simulink model "rectifire_single_inverter_pv1"  (R2022b)
settings: Solver=ode23tb  StartTime=0  StopTime=3  RelTol=1e-4
undefined symbols (not defined in the file): Ion, Lithium, P_100, sigbuilder_block, time_step
libraries: spsSeriesRLCBranchLib x26, spsTriangleGeneratorLib x26, slpidlib x26, spsVoltageMeasurementLib x14, spsCurrentMeasurementLib x11, spsDiodeLib x9, simulink x8, spsIGBTDiodeLib x8, spsMosfetLib x8, powerlib_extras x4, spsGroundLib x2, spsBatteryLib x2
(part 3 of 6)

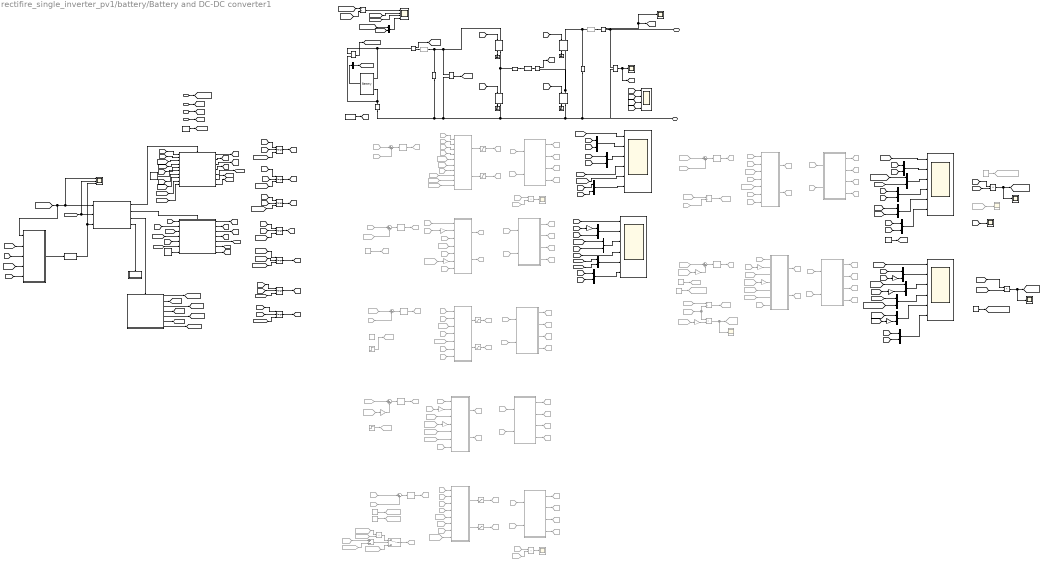
== system rectifire_single_inverter_pv1/battery/Battery and DC-DC converter1 ==
  note: Discharge in Constant Power Mode : realize by constant current
  note: Be charged in constant Current Mode
  note: Discharge in constant Current Mode
  note: Discharge in constant Voltage Mode
  note: 和开关频率同步
  note: FSBB Passivity Based Control
      | control algorithm ref: https://www.youtube.com/watch?v=5YT7cERlMrg
      | 1. Modify the topology corresponding to Gosspower hardware.
      | 1.1 add additional capacities in both input and output side
      | 1.2 add additional 2.2e-6H inductor in both input and output side to mitigate the fluctuation in constant current mode.
      | 2. Realize the constant current/voltage/Power mode in charge/discharge mode.
      |
      | Author LokiXun rongji.xun@gmail.com
  note: Be Charged in constant Voltage Mode
  note: Be Charged in Constant Power Mode : realize by constant current
  note: Constant Current/Power Transition Point
  note: Discharge in Constant Current Mode using Voltage control
  note: Charge Mode
  note: Discharge Mode
  note: Current/Voltage Protection
  Mode=Charge0/DIscharge1 : Inport
  battery_I_charge_ref : Inport  Port=2
  V_bus_ref : Inport  Port=3
  Bus_load : Inport  Port=4
  "85 volts, 100 Ah LithiumIon battery " : spsBatteryLib/Battery  BatType=Lithium-Ion  ShowTempParam=off  ThermalPreset=no  ShowAgeParam=off  NomV=85  NomQ=100  SOC=20  Batt_Tr=30  PresetModel=off  MaxQ=107.6923  MinV=83.2  FullV=115.2  Dis_rate=43.4783  R=0.08  Normal_OP=96.1538  expZone=[92.2034, 20]  current=[6.5 13 32.5]  Units=Time  Tci=20  NomT=20  T2=-30  MaxQ2=4.8  FullV2=7.1  Normal_OP2=5.655  expZone2="[6.58           1]"  Rca=0.6  ti=2000  Dp=0  Neq0=0  Tsim=1e6  Ta1=25  Qeol=5.4*0.9  Reol=0.013333*1.2  Char_age=[2.3478, 3]  Dis_age=[2.3478, 10]  N1=1500  N2=10500  N3=1000  N4=1400  Ta2=45  N5=950
      settings: LibrarySourceBlock=electricdrivelib/Extra Sources/Battery
  ActualPower1 : Scope  Commented=on
  ActualPower2 : Scope
  Battery Load : Scope  NumInputPorts=4
  BatteryCurrent1 : Scope  Commented=on
  Bus Selector : BusSelector  OutputSignals=SOC (%)
  BusPower : Scope
  C1 : spsSeriesRLCBranchLib/Series RLC Branch  LConnTagsString=__new0  RConnTagsString=__new0  BranchType=C  Resistance=0.01  Inductance=1e-3  SetiL0=off  InitialCurrent=0  Capacitance=1440e-6  Setx0=on  InitialVoltage=90  Measurements=None
  C2 : spsSeriesRLCBranchLib/Series RLC Branch  LConnTagsString=__new0  RConnTagsString=__new0  BranchType=C  Resistance=5  Inductance=1e-3  SetiL0=off  InitialCurrent=0  Capacitance=1440e-6  Setx0=on  InitialVoltage=90  Measurements=None
  Cast To Double : DataTypeConversion  OutDataTypeStr=double  SaturateOnIntegerOverflow=off  RndMeth=Floor
  Charge : Scope  NumInputPorts=6
  Charge Mixed CurrentPower1 : Subsystem  TreatAsAtomicUnit=on
  Charge Mixed CurrentPower2 : Subsystem  TreatAsAtomicUnit=on
  Constant1 : Constant  Value=time_step
  Constant10 : Constant  Value=3000
  Constant11 : Constant  Commented=on  Value=96
  Constant12 : Constant  Commented=on  Value=101
  Constant14 : Constant  Commented=on  Value=103.5
  Constant16 : Constant  Value=101
  Constant20 : Constant  Commented=on  Value=100
  Constant3 : Constant  Commented=on  Value=26
  Constant4 : Constant  Commented=on  Value=29
  Constant5 : Constant  Commented=on  Value=3000
  Current Measurement : spsCurrentMeasurementLib/Current Measurement  PhasorSimulation=off  OutputType=Complex  PSBequivalent=0
  Current Measurement1 : spsCurrentMeasurementLib/Current Measurement  PhasorSimulation=off  OutputType=Complex  PSBequivalent=0
  DM_inductor1 : spsSeriesRLCBranchLib/Series RLC Branch  Commented=through  LConnTagsString=__new0  RConnTagsString=__new0  BranchType=L  Resistance=1.0  Inductance=2.2e-6  SetiL0=off  InitialCurrent=0  Capacitance=1.0  Setx0=off  InitialVoltage=0  Measurements=None
  DM_inductor2 : spsSeriesRLCBranchLib/Series RLC Branch  Commented=through  LConnTagsString=__new0  RConnTagsString=__new0  BranchType=L  Resistance=1.0  Inductance=2.2e-6  SetiL0=off  InitialCurrent=0  Capacitance=1.0  Setx0=off  InitialVoltage=0  Measurements=None
  Discharge : Scope  NumInputPorts=6
  Discharge Const Voltage : Subsystem  TreatAsAtomicUnit=on
  Discharge+V : Scope  NumInputPorts=6
  Divide : Product  Commented=on  Inputs=*/
  Divide1 : Product  Commented=on  Inputs=*/
  Divide3 : Product  Inputs=*/
  DoNothing2 : Subsystem  TreatAsAtomicUnit=on
  From{10,24,30,32,152,168,190} (7 alike) : From  Commented=on  GotoTag=iL
  From{37..38,57..58,101,172,174,202} (8 alike) : From  Commented=on  GotoTag=i_out_ref
  From103 : From  Commented=on  GotoTag=Power_ref
  From{14,33,59,77,94,104,155,169,203} (9 alike) : From  Commented=on  GotoTag=V_battery
  From{34,41,60,74,95,107,197..198} (8 alike) : From  Commented=on  GotoTag=i_battery
  From{11..12,45,70,75,153} (6 alike) : From  Commented=on  GotoTag=VC_ref
  From{8,13,28,52..53,76,88,98,154,189,191,199} (12 alike) : From  Commented=on  GotoTag=V_bus
  From148 : From  Commented=on  GotoTag=Bus_load
  From156 : From  Commented=on  GotoTag=Bus_load
  From{18,35,54,78,157,170,200} (7 alike) : From  Commented=on  GotoTag=Ts
  From{9,36,56,79,158,171,201} (7 alike) : From  Commented=on  GotoTag=iL_ref
  From{29,31,46,55,92,96,159,192..193} (9 alike) : From  Commented=on  GotoTag=i_out
  From{16,39,49,61,64,80,173} (7 alike) : From  Commented=on  GotoTag=u1
  From{17,40,50,62,81,93,175} (7 alike) : From  Commented=on  GotoTag=u2
  From188 : From  Commented=on  GotoTag=Power_ref
  From43 : From  Commented=on  GotoTag=Power_max
  From44 : From  Commented=on  GotoTag=i_out_max_ref
  From47 : From  Commented=on  GotoTag=V_out_initial
  From48 : From  Commented=on  GotoTag=i_out_max_ref
  From51 : From  Commented=on  GotoTag=Bus_load
  Gain{,2..3,6,10..12,16..17} (9 alike) : Gain  Commented=on  Gain=-1
  Gain{7..8,14..15} (4 alike) : Gain  Gain=-1
  Goto{10,21,28..29,34,42,92} (7 alike) : Goto  Commented=on  GotoTag=S4
  Goto100 : Goto  Commented=on  GotoTag=V_power_starup
  Goto{6,12,15,17,81,88,101} (7 alike) : Goto  Commented=on  GotoTag=u1
  Goto{7,14,18,25,89,102,119} (7 alike) : Goto  Commented=on  GotoTag=u2
  Goto{8,23,31,40,77,94,103} (7 alike) : Goto  Commented=on  GotoTag=S1
  Goto{9,24,32,41,78,95,104} (7 alike) : Goto  Commented=on  GotoTag=S3
  Goto{11,22,30,33,35,43,93} (7 alike) : Goto  Commented=on  GotoTag=S2
  Goto120 : Goto  Commented=on  GotoTag=V_out_initial
  Goto126 : Goto  Commented=on  GotoTag=V_discharge_PowerMode
  Goto{19,26,46,96} (4 alike) : Goto  Commented=on  GotoTag=i_out_ref
  Goto{2,20,27,36,39,75,91} (7 alike) : Goto  Commented=on  GotoTag=iL_ref
  Goto37 : Goto  Commented=on  GotoTag=VC_ref
  Goto38 : Goto  Commented=on  GotoTag=Power_ref
  Goto76 : Goto  Commented=on  GotoTag=VC_ref
  Goto80 : Goto  Commented=on  GotoTag=i_out_max_ref
  Goto99 : Goto  Commented=on  GotoTag=Power_out
  IGBT/Diode{1..4} (4 alike) : spsIGBTDiodeLib/IGBT//Diode  Ron=1e-3  Rs=1e5  Cs=inf  Measurements=on
  IL6 : spsCurrentMeasurementLib/Current Measurement  PhasorSimulation=off  OutputType=Complex  PSBequivalent=0
  I_bus_scope : Scope
  If1 : If  NumInputs=3  IfExpression="u3 == 0 & u1 == 1  & u2 > 10"  ElseIfExpressions=u3 == 0 & u1 == 0 & u2 < 95, u3==1
  MATLAB Function : MATLAB Function  Commented=on  TreatAsAtomicUnit=on
  MATLAB Function1 : MATLAB Function  Commented=on  TreatAsAtomicUnit=on
  MATLAB Function2 : MATLAB Function  Commented=on  TreatAsAtomicUnit=on
  MATLAB Function3 : MATLAB Function  Commented=on  TreatAsAtomicUnit=on
  MATLAB Function4 : MATLAB Function  TreatAsAtomicUnit=on
  MATLAB Function5 : MATLAB Function  Commented=on  TreatAsAtomicUnit=on
  MATLAB Function6 : MATLAB Function  Commented=on  TreatAsAtomicUnit=on
  MATLAB Function7 : MATLAB Function  Commented=on  TreatAsAtomicUnit=on
  Minus : Sum  Commented=on  Inputs=+-
  Modulation : Subsystem  Commented=on
  Modulation1 : Subsystem  Commented=on
  Modulation2 : Subsystem  Commented=on
  Modulation3 : Subsystem  Commented=on
  Modulation4 : Subsystem  Commented=on
  Modulation5 : Subsystem  Commented=on
  Modulation6 : Subsystem  Commented=on
  Mux{,1..4,9..21} (18 alike) : Mux  Inputs=2
  PID Controller1 : slpidlib/PID Controller  Commented=on  Controller=PI  Form=Parallel  TimeDomain=Continuous-time  UseExternalTs=off  SampleTime=-1  IntegratorMethod=Forward Euler  FilterMethod=Forward Euler  ControllerParametersSource=internal  P=6.7500  I=8.1000e+03 * 2  UseKiTs=on  D=0  N=100  UseFilter=on  TunerSelectOption=Transfer Function Based (PID Tuner App)  InitialConditionSource=internal  InitialConditionForIntegrator=0  InitialConditionForFilter=0  DifferentiatorICPrevScaledInput=0  ExternalReset=none  TrackingMode=off  Kt=1  LimitOutput=on  SatLimitsSource=internal  UpperSaturationLimit=50  LowerSaturationLimit=-10  LinearizeAsGain=on  AntiWindupMode=none  Kb=1  LimitIntegrator=off  UpperIntegratorSaturationLimit=inf  LowerIntegratorSaturationLimit=-inf  POutMin=[]  POutMax=[]  IOutMin=[]  IOutMax=[]  DOutMin=[]  DOutMax=[]  NOutMin=[]  NOutMax=[]  SumOutMin=[]  SumOutMax=[]  SaturationOutMin=[]  SaturationOutMax=[]  PParamMin=[]  PParamMax=[]  IParamMin=[]  IParamMax=[]  DParamMin=[]  DParamMax=[]  NParamMin=[]  NParamMax=[]  KbParamMin=[]  KbParamMax=[]  KtParamMin=[]  KtParamMax=[]  KbOutMin=[]  KbOutMax=[]  KtOutMin=[]  KtOutMax=[]  IntegratorOutMin=[]  IntegratorOutMax=[]  FilterOutMin=[]  FilterOutMax=[]  SumI1OutMin=[]  SumI1OutMax=[]  SumI2OutMin=[]  SumI2OutMax=[]  SumI3OutMin=[]  SumI3OutMax=[]  SumI4OutMin=[]  SumI4OutMax=[]  SumDOutMin=[]  SumDOutMax=[]  DifferentiatorOutMin=[]  DifferentiatorOutMax=[]  FilterDiffOutCoefMin=[]  FilterDiffOutCoefMax=[]  ReciprocalOutMin=[]  ReciprocalOutMax=[]  SumDenOutMin=[]  SumDenOutMax=[]  SumNumOutMin=[]  SumNumOutMax=[]  DivideOutMin=[]  DivideOutMax=[]  UdiffTsProdOutMin=[]  UdiffTsProdOutMax=[]  NTsProdOutMin=[]  NTsProdOutMax=[]  UintegralTsProdOutMin=[]  UintegralTsProdOutMax=[]  UngainTsProdOutMin=[]  UngainTsProdOutMax=[]  ClampingZeroOutDataTypeStr=Inherit: Inherit via back propagation  ClampingZeroOutMin=[]  ClampingZeroOutMax=[]  FilterDenConstantOutDataTypeStr=Inherit: Inherit via back propagation  FilterDenConstantOutMin=[]  FilterDenConstantOutMax=[]  PCopyOutDataTypeStr=Inherit: Inherit via back propagation  PCopyOutMin=[]  PCopyOutMax=[]  NCopyOutDataTypeStr=Inherit: Inherit via back propagation  NCopyOutMin=[]  NCopyOutMax=[]  IntegratorContinuousStateAttributes=''  IntegratorStateMustResolveToSignalObject=off  IntegratorRTWStateStorageClass=Auto  FilterContinuousStateAttributes=''  FilterStateMustResolveToSignalObject=off  FilterRTWStateStorageClass=Auto  ParallelPVariant=InternalParameters  IdealPVariant=Disabled  IVariant=InternalParameters  DVariant=Disabled  IntegratorVariant=Continuous  SatVariant=Enabled  AWVariant=Passthrough  PCopyVariant=Disabled  TRVariant=Disabled  FdbkBlocksVariant=Forward  IdealPFdbkVariant=Disabled  SatFdbkVariant=Disabled  DerivativeFilterVariant=Disabled  NVariant=Disabled  NCopyVariant=Disabled_SignalSpec  FilterICVariant=Disabled  IntegratorICVariant=InternalICs  ExternalResetVariant=Disabled  TRSumVariant=Passthrough  SumFdbkVariant=Disabled  SumVariant=Sum_PI  TsampFilterVariant=InternalTs  TsampNgainVariant=Passthrough  TsampIntegralVariant=Passthrough  ExternalSaturationOutDataTypeStr=Inherit: Same as second input
  PID Controller2 : slpidlib/PID Controller  Commented=on  Controller=PI  Form=Parallel  TimeDomain=Continuous-time  UseExternalTs=off  SampleTime=-1  IntegratorMethod=Forward Euler  FilterMethod=Forward Euler  ControllerParametersSource=internal  P=45 * 2  I=1.3361e+05 /25  UseKiTs=on  D=0  N=100  UseFilter=on  TunerSelectOption=Frequency Response Based  InitialConditionSource=internal  InitialConditionForIntegrator=0  InitialConditionForFilter=0  DifferentiatorICPrevScaledInput=0  ExternalReset=none  TrackingMode=off  Kt=1  LimitOutput=on  SatLimitsSource=internal  UpperSaturationLimit=50  LowerSaturationLimit=-10  LinearizeAsGain=on  AntiWindupMode=none  Kb=1  LimitIntegrator=off  UpperIntegratorSaturationLimit=inf  LowerIntegratorSaturationLimit=-inf  POutMin=[]  POutMax=[]  IOutMin=[]  IOutMax=[]  DOutMin=[]  DOutMax=[]  NOutMin=[]  NOutMax=[]  SumOutMin=[]  SumOutMax=[]  SaturationOutMin=[]  SaturationOutMax=[]  PParamMin=[]  PParamMax=[]  IParamMin=[]  IParamMax=[]  DParamMin=[]  DParamMax=[]  NParamMin=[]  NParamMax=[]  KbParamMin=[]  KbParamMax=[]  KtParamMin=[]  KtParamMax=[]  KbOutMin=[]  KbOutMax=[]  KtOutMin=[]  KtOutMax=[]  IntegratorOutMin=[]  IntegratorOutMax=[]  FilterOutMin=[]  FilterOutMax=[]  SumI1OutMin=[]  SumI1OutMax=[]  SumI2OutMin=[]  SumI2OutMax=[]  SumI3OutMin=[]  SumI3OutMax=[]  SumI4OutMin=[]  SumI4OutMax=[]  SumDOutMin=[]  SumDOutMax=[]  DifferentiatorOutMin=[]  DifferentiatorOutMax=[]  FilterDiffOutCoefMin=[]  FilterDiffOutCoefMax=[]  ReciprocalOutMin=[]  ReciprocalOutMax=[]  SumDenOutMin=[]  SumDenOutMax=[]  SumNumOutMin=[]  SumNumOutMax=[]  DivideOutMin=[]  DivideOutMax=[]  UdiffTsProdOutMin=[]  UdiffTsProdOutMax=[]  NTsProdOutMin=[]  NTsProdOutMax=[]  UintegralTsProdOutMin=[]  UintegralTsProdOutMax=[]  UngainTsProdOutMin=[]  UngainTsProdOutMax=[]  ClampingZeroOutDataTypeStr=Inherit: Inherit via back propagation  ClampingZeroOutMin=[]  ClampingZeroOutMax=[]  FilterDenConstantOutDataTypeStr=Inherit: Inherit via back propagation  FilterDenConstantOutMin=[]  FilterDenConstantOutMax=[]  PCopyOutDataTypeStr=Inherit: Inherit via back propagation  PCopyOutMin=[]  PCopyOutMax=[]  NCopyOutDataTypeStr=Inherit: Inherit via back propagation  NCopyOutMin=[]  NCopyOutMax=[]  IntegratorContinuousStateAttributes=''  IntegratorStateMustResolveToSignalObject=off  IntegratorRTWStateStorageClass=Auto  FilterContinuousStateAttributes=''  FilterStateMustResolveToSignalObject=off  FilterRTWStateStorageClass=Auto  ParallelPVariant=InternalParameters  IdealPVariant=Disabled  IVariant=InternalParameters  DVariant=Disabled  IntegratorVariant=Continuous  SatVariant=Enabled  AWVariant=Passthrough  PCopyVariant=Disabled  TRVariant=Disabled  FdbkBlocksVariant=Forward  IdealPFdbkVariant=Disabled  SatFdbkVariant=Disabled  DerivativeFilterVariant=Disabled  NVariant=Disabled  NCopyVariant=Disabled_SignalSpec  FilterICVariant=Disabled  IntegratorICVariant=InternalICs  ExternalResetVariant=Disabled  TRSumVariant=Passthrough  SumFdbkVariant=Disabled  SumVariant=Sum_PI  TsampFilterVariant=InternalTs  TsampNgainVariant=Passthrough  TsampIntegralVariant=Passthrough  ExternalSaturationOutDataTypeStr=Inherit: Same as second input
  PID Controller3 : slpidlib/PID Controller  Commented=on  Controller=PI  Form=Parallel  TimeDomain=Continuous-time  UseExternalTs=off  SampleTime=-1  IntegratorMethod=Forward Euler  FilterMethod=Forward Euler  ControllerParametersSource=internal  P=6.7500  I=8.1000e+03 * 2  UseKiTs=on  D=0  N=100  UseFilter=on  TunerSelectOption=Transfer Function Based (PID Tuner App)  InitialConditionSource=internal  InitialConditionForIntegrator=0  InitialConditionForFilter=0  DifferentiatorICPrevScaledInput=0  ExternalReset=none  TrackingMode=off  Kt=1  LimitOutput=on  SatLimitsSource=internal  UpperSaturationLimit=50  LowerSaturationLimit=-10  LinearizeAsGain=on  AntiWindupMode=none  Kb=1  LimitIntegrator=off  UpperIntegratorSaturationLimit=inf  LowerIntegratorSaturationLimit=-inf  POutMin=[]  POutMax=[]  IOutMin=[]  IOutMax=[]  DOutMin=[]  DOutMax=[]  NOutMin=[]  NOutMax=[]  SumOutMin=[]  SumOutMax=[]  SaturationOutMin=[]  SaturationOutMax=[]  PParamMin=[]  PParamMax=[]  IParamMin=[]  IParamMax=[]  DParamMin=[]  DParamMax=[]  NParamMin=[]  NParamMax=[]  KbParamMin=[]  KbParamMax=[]  KtParamMin=[]  KtParamMax=[]  KbOutMin=[]  KbOutMax=[]  KtOutMin=[]  KtOutMax=[]  IntegratorOutMin=[]  IntegratorOutMax=[]  FilterOutMin=[]  FilterOutMax=[]  SumI1OutMin=[]  SumI1OutMax=[]  SumI2OutMin=[]  SumI2OutMax=[]  SumI3OutMin=[]  SumI3OutMax=[]  SumI4OutMin=[]  SumI4OutMax=[]  SumDOutMin=[]  SumDOutMax=[]  DifferentiatorOutMin=[]  DifferentiatorOutMax=[]  FilterDiffOutCoefMin=[]  FilterDiffOutCoefMax=[]  ReciprocalOutMin=[]  ReciprocalOutMax=[]  SumDenOutMin=[]  SumDenOutMax=[]  SumNumOutMin=[]  SumNumOutMax=[]  DivideOutMin=[]  DivideOutMax=[]  UdiffTsProdOutMin=[]  UdiffTsProdOutMax=[]  NTsProdOutMin=[]  NTsProdOutMax=[]  UintegralTsProdOutMin=[]  UintegralTsProdOutMax=[]  UngainTsProdOutMin=[]  UngainTsProdOutMax=[]  ClampingZeroOutDataTypeStr=Inherit: Inherit via back propagation  ClampingZeroOutMin=[]  ClampingZeroOutMax=[]  FilterDenConstantOutDataTypeStr=Inherit: Inherit via back propagation  FilterDenConstantOutMin=[]  FilterDenConstantOutMax=[]  PCopyOutDataTypeStr=Inherit: Inherit via back propagation  PCopyOutMin=[]  PCopyOutMax=[]  NCopyOutDataTypeStr=Inherit: Inherit via back propagation  NCopyOutMin=[]  NCopyOutMax=[]  IntegratorContinuousStateAttributes=''  IntegratorStateMustResolveToSignalObject=off  IntegratorRTWStateStorageClass=Auto  FilterContinuousStateAttributes=''  FilterStateMustResolveToSignalObject=off  FilterRTWStateStorageClass=Auto  ParallelPVariant=InternalParameters  IdealPVariant=Disabled  IVariant=InternalParameters  DVariant=Disabled  IntegratorVariant=Continuous  SatVariant=Enabled  AWVariant=Passthrough  PCopyVariant=Disabled  TRVariant=Disabled  FdbkBlocksVariant=Forward  IdealPFdbkVariant=Disabled  SatFdbkVariant=Disabled  DerivativeFilterVariant=Disabled  NVariant=Disabled  NCopyVariant=Disabled_SignalSpec  FilterICVariant=Disabled  IntegratorICVariant=InternalICs  ExternalResetVariant=Disabled  TRSumVariant=Passthrough  SumFdbkVariant=Disabled  SumVariant=Sum_PI  TsampFilterVariant=InternalTs  TsampNgainVariant=Passthrough  TsampIntegralVariant=Passthrough  ExternalSaturationOutDataTypeStr=Inherit: Same as second input
  PID Controller4 : slpidlib/PID Controller  Commented=on  Controller=PI  Form=Parallel  TimeDomain=Continuous-time  UseExternalTs=off  SampleTime=-1  IntegratorMethod=Forward Euler  FilterMethod=Forward Euler  ControllerParametersSource=internal  P=15  I=1000  UseKiTs=on  D=0  N=100  UseFilter=on  TunerSelectOption=Transfer Function Based (PID Tuner App)  InitialConditionSource=internal  InitialConditionForIntegrator=0  InitialConditionForFilter=0  DifferentiatorICPrevScaledInput=0  ExternalReset=none  TrackingMode=off  Kt=1  LimitOutput=on  SatLimitsSource=internal  UpperSaturationLimit=50  LowerSaturationLimit=-10  LinearizeAsGain=on  AntiWindupMode=none  Kb=1  LimitIntegrator=off  UpperIntegratorSaturationLimit=inf  LowerIntegratorSaturationLimit=-inf  POutMin=[]  POutMax=[]  IOutMin=[]  IOutMax=[]  DOutMin=[]  DOutMax=[]  NOutMin=[]  NOutMax=[]  SumOutMin=[]  SumOutMax=[]  SaturationOutMin=[]  SaturationOutMax=[]  PParamMin=[]  PParamMax=[]  IParamMin=[]  IParamMax=[]  DParamMin=[]  DParamMax=[]  NParamMin=[]  NParamMax=[]  KbParamMin=[]  KbParamMax=[]  KtParamMin=[]  KtParamMax=[]  KbOutMin=[]  KbOutMax=[]  KtOutMin=[]  KtOutMax=[]  IntegratorOutMin=[]  IntegratorOutMax=[]  FilterOutMin=[]  FilterOutMax=[]  SumI1OutMin=[]  SumI1OutMax=[]  SumI2OutMin=[]  SumI2OutMax=[]  SumI3OutMin=[]  SumI3OutMax=[]  SumI4OutMin=[]  SumI4OutMax=[]  SumDOutMin=[]  SumDOutMax=[]  DifferentiatorOutMin=[]  DifferentiatorOutMax=[]  FilterDiffOutCoefMin=[]  FilterDiffOutCoefMax=[]  ReciprocalOutMin=[]  ReciprocalOutMax=[]  SumDenOutMin=[]  SumDenOutMax=[]  SumNumOutMin=[]  SumNumOutMax=[]  DivideOutMin=[]  DivideOutMax=[]  UdiffTsProdOutMin=[]  UdiffTsProdOutMax=[]  NTsProdOutMin=[]  NTsProdOutMax=[]  UintegralTsProdOutMin=[]  UintegralTsProdOutMax=[]  UngainTsProdOutMin=[]  UngainTsProdOutMax=[]  ClampingZeroOutDataTypeStr=Inherit: Inherit via back propagation  ClampingZeroOutMin=[]  ClampingZeroOutMax=[]  FilterDenConstantOutDataTypeStr=Inherit: Inherit via back propagation  FilterDenConstantOutMin=[]  FilterDenConstantOutMax=[]  PCopyOutDataTypeStr=Inherit: Inherit via back propagation  PCopyOutMin=[]  PCopyOutMax=[]  NCopyOutDataTypeStr=Inherit: Inherit via back propagation  NCopyOutMin=[]  NCopyOutMax=[]  IntegratorContinuousStateAttributes=''  IntegratorStateMustResolveToSignalObject=off  IntegratorRTWStateStorageClass=Auto  FilterContinuousStateAttributes=''  FilterStateMustResolveToSignalObject=off  FilterRTWStateStorageClass=Auto  ParallelPVariant=InternalParameters  IdealPVariant=Disabled  IVariant=InternalParameters  DVariant=Disabled  IntegratorVariant=Continuous  SatVariant=Enabled  AWVariant=Passthrough  PCopyVariant=Disabled  TRVariant=Disabled  FdbkBlocksVariant=Forward  IdealPFdbkVariant=Disabled  SatFdbkVariant=Disabled  DerivativeFilterVariant=Disabled  NVariant=Disabled  NCopyVariant=Disabled_SignalSpec  FilterICVariant=Disabled  IntegratorICVariant=InternalICs  ExternalResetVariant=Disabled  TRSumVariant=Passthrough  SumFdbkVariant=Disabled  SumVariant=Sum_PI  TsampFilterVariant=InternalTs  TsampNgainVariant=Passthrough  TsampIntegralVariant=Passthrough  ExternalSaturationOutDataTypeStr=Inherit: Same as second input
  PID Controller5 : slpidlib/PID Controller  Commented=on  Controller=PI  Form=Parallel  TimeDomain=Continuous-time  UseExternalTs=off  SampleTime=-1  IntegratorMethod=Forward Euler  FilterMethod=Forward Euler  ControllerParametersSource=internal  P=15  I=1000  UseKiTs=on  D=0  N=100  UseFilter=on  TunerSelectOption=Transfer Function Based (PID Tuner App)  InitialConditionSource=internal  InitialConditionForIntegrator=0  InitialConditionForFilter=0  DifferentiatorICPrevScaledInput=0  ExternalReset=none  TrackingMode=off  Kt=1  LimitOutput=on  SatLimitsSource=internal  UpperSaturationLimit=50  LowerSaturationLimit=-10  LinearizeAsGain=on  AntiWindupMode=none  Kb=1  LimitIntegrator=off  UpperIntegratorSaturationLimit=inf  LowerIntegratorSaturationLimit=-inf  POutMin=[]  POutMax=[]  IOutMin=[]  IOutMax=[]  DOutMin=[]  DOutMax=[]  NOutMin=[]  NOutMax=[]  SumOutMin=[]  SumOutMax=[]  SaturationOutMin=[]  SaturationOutMax=[]  PParamMin=[]  PParamMax=[]  IParamMin=[]  IParamMax=[]  DParamMin=[]  DParamMax=[]  NParamMin=[]  NParamMax=[]  KbParamMin=[]  KbParamMax=[]  KtParamMin=[]  KtParamMax=[]  KbOutMin=[]  KbOutMax=[]  KtOutMin=[]  KtOutMax=[]  IntegratorOutMin=[]  IntegratorOutMax=[]  FilterOutMin=[]  FilterOutMax=[]  SumI1OutMin=[]  SumI1OutMax=[]  SumI2OutMin=[]  SumI2OutMax=[]  SumI3OutMin=[]  SumI3OutMax=[]  SumI4OutMin=[]  SumI4OutMax=[]  SumDOutMin=[]  SumDOutMax=[]  DifferentiatorOutMin=[]  DifferentiatorOutMax=[]  FilterDiffOutCoefMin=[]  FilterDiffOutCoefMax=[]  ReciprocalOutMin=[]  ReciprocalOutMax=[]  SumDenOutMin=[]  SumDenOutMax=[]  SumNumOutMin=[]  SumNumOutMax=[]  DivideOutMin=[]  DivideOutMax=[]  UdiffTsProdOutMin=[]  UdiffTsProdOutMax=[]  NTsProdOutMin=[]  NTsProdOutMax=[]  UintegralTsProdOutMin=[]  UintegralTsProdOutMax=[]  UngainTsProdOutMin=[]  UngainTsProdOutMax=[]  ClampingZeroOutDataTypeStr=Inherit: Inherit via back propagation  ClampingZeroOutMin=[]  ClampingZeroOutMax=[]  FilterDenConstantOutDataTypeStr=Inherit: Inherit via back propagation  FilterDenConstantOutMin=[]  FilterDenConstantOutMax=[]  PCopyOutDataTypeStr=Inherit: Inherit via back propagation  PCopyOutMin=[]  PCopyOutMax=[]  NCopyOutDataTypeStr=Inherit: Inherit via back propagation  NCopyOutMin=[]  NCopyOutMax=[]  IntegratorContinuousStateAttributes=''  IntegratorStateMustResolveToSignalObject=off  IntegratorRTWStateStorageClass=Auto  FilterContinuousStateAttributes=''  FilterStateMustResolveToSignalObject=off  FilterRTWStateStorageClass=Auto  ParallelPVariant=InternalParameters  IdealPVariant=Disabled  IVariant=InternalParameters  DVariant=Disabled  IntegratorVariant=Continuous  SatVariant=Enabled  AWVariant=Passthrough  PCopyVariant=Disabled  TRVariant=Disabled  FdbkBlocksVariant=Forward  IdealPFdbkVariant=Disabled  SatFdbkVariant=Disabled  DerivativeFilterVariant=Disabled  NVariant=Disabled  NCopyVariant=Disabled_SignalSpec  FilterICVariant=Disabled  IntegratorICVariant=InternalICs  ExternalResetVariant=Disabled  TRSumVariant=Passthrough  SumFdbkVariant=Disabled  SumVariant=Sum_PI  TsampFilterVariant=InternalTs  TsampNgainVariant=Passthrough  TsampIntegralVariant=Passthrough  ExternalSaturationOutDataTypeStr=Inherit: Same as second input
  PID Controller6 : slpidlib/PID Controller  Commented=on  Controller=PI  Form=Parallel  TimeDomain=Continuous-time  UseExternalTs=off  SampleTime=-1  IntegratorMethod=Forward Euler  FilterMethod=Forward Euler  ControllerParametersSource=internal  P=15  I=1000  UseKiTs=on  D=0  N=100  UseFilter=on  TunerSelectOption=Transfer Function Based (PID Tuner App)  InitialConditionSource=internal  InitialConditionForIntegrator=0  InitialConditionForFilter=0  DifferentiatorICPrevScaledInput=0  ExternalReset=none  TrackingMode=off  Kt=1  LimitOutput=on  SatLimitsSource=internal  UpperSaturationLimit=50  LowerSaturationLimit=-10  LinearizeAsGain=on  AntiWindupMode=none  Kb=1  LimitIntegrator=off  UpperIntegratorSaturationLimit=inf  LowerIntegratorSaturationLimit=-inf  POutMin=[]  POutMax=[]  IOutMin=[]  IOutMax=[]  DOutMin=[]  DOutMax=[]  NOutMin=[]  NOutMax=[]  SumOutMin=[]  SumOutMax=[]  SaturationOutMin=[]  SaturationOutMax=[]  PParamMin=[]  PParamMax=[]  IParamMin=[]  IParamMax=[]  DParamMin=[]  DParamMax=[]  NParamMin=[]  NParamMax=[]  KbParamMin=[]  KbParamMax=[]  KtParamMin=[]  KtParamMax=[]  KbOutMin=[]  KbOutMax=[]  KtOutMin=[]  KtOutMax=[]  IntegratorOutMin=[]  IntegratorOutMax=[]  FilterOutMin=[]  FilterOutMax=[]  SumI1OutMin=[]  SumI1OutMax=[]  SumI2OutMin=[]  SumI2OutMax=[]  SumI3OutMin=[]  SumI3OutMax=[]  SumI4OutMin=[]  SumI4OutMax=[]  SumDOutMin=[]  SumDOutMax=[]  DifferentiatorOutMin=[]  DifferentiatorOutMax=[]  FilterDiffOutCoefMin=[]  FilterDiffOutCoefMax=[]  ReciprocalOutMin=[]  ReciprocalOutMax=[]  SumDenOutMin=[]  SumDenOutMax=[]  SumNumOutMin=[]  SumNumOutMax=[]  DivideOutMin=[]  DivideOutMax=[]  UdiffTsProdOutMin=[]  UdiffTsProdOutMax=[]  NTsProdOutMin=[]  NTsProdOutMax=[]  UintegralTsProdOutMin=[]  UintegralTsProdOutMax=[]  UngainTsProdOutMin=[]  UngainTsProdOutMax=[]  ClampingZeroOutDataTypeStr=Inherit: Inherit via back propagation  ClampingZeroOutMin=[]  ClampingZeroOutMax=[]  FilterDenConstantOutDataTypeStr=Inherit: Inherit via back propagation  FilterDenConstantOutMin=[]  FilterDenConstantOutMax=[]  PCopyOutDataTypeStr=Inherit: Inherit via back propagation  PCopyOutMin=[]  PCopyOutMax=[]  NCopyOutDataTypeStr=Inherit: Inherit via back propagation  NCopyOutMin=[]  NCopyOutMax=[]  IntegratorContinuousStateAttributes=''  IntegratorStateMustResolveToSignalObject=off  IntegratorRTWStateStorageClass=Auto  FilterContinuousStateAttributes=''  FilterStateMustResolveToSignalObject=off  FilterRTWStateStorageClass=Auto  ParallelPVariant=InternalParameters  IdealPVariant=Disabled  IVariant=InternalParameters  DVariant=Disabled  IntegratorVariant=Continuous  SatVariant=Enabled  AWVariant=Passthrough  PCopyVariant=Disabled  TRVariant=Disabled  FdbkBlocksVariant=Forward  IdealPFdbkVariant=Disabled  SatFdbkVariant=Disabled  DerivativeFilterVariant=Disabled  NVariant=Disabled  NCopyVariant=Disabled_SignalSpec  FilterICVariant=Disabled  IntegratorICVariant=InternalICs  ExternalResetVariant=Disabled  TRSumVariant=Passthrough  SumFdbkVariant=Disabled  SumVariant=Sum_PI  TsampFilterVariant=InternalTs  TsampNgainVariant=Passthrough  TsampIntegralVariant=Passthrough  ExternalSaturationOutDataTypeStr=Inherit: Same as second input
  PID Controller7 : slpidlib/PID Controller  Commented=on  Controller=PI  Form=Parallel  TimeDomain=Continuous-time  UseExternalTs=off  SampleTime=-1  IntegratorMethod=Forward Euler  FilterMethod=Forward Euler  ControllerParametersSource=internal  P=45 * 2  I=1.3361e+05 /25  UseKiTs=on  D=0  N=100  UseFilter=on  TunerSelectOption=Transfer Function Based (PID Tuner App)  InitialConditionSource=internal  InitialConditionForIntegrator=0  InitialConditionForFilter=0  DifferentiatorICPrevScaledInput=0  ExternalReset=none  TrackingMode=off  Kt=1  LimitOutput=on  SatLimitsSource=internal  UpperSaturationLimit=50  LowerSaturationLimit=-10  LinearizeAsGain=on  AntiWindupMode=none  Kb=1  LimitIntegrator=off  UpperIntegratorSaturationLimit=inf  LowerIntegratorSaturationLimit=-inf  POutMin=[]  POutMax=[]  IOutMin=[]  IOutMax=[]  DOutMin=[]  DOutMax=[]  NOutMin=[]  NOutMax=[]  SumOutMin=[]  SumOutMax=[]  SaturationOutMin=[]  SaturationOutMax=[]  PParamMin=[]  PParamMax=[]  IParamMin=[]  IParamMax=[]  DParamMin=[]  DParamMax=[]  NParamMin=[]  NParamMax=[]  KbParamMin=[]  KbParamMax=[]  KtParamMin=[]  KtParamMax=[]  KbOutMin=[]  KbOutMax=[]  KtOutMin=[]  KtOutMax=[]  IntegratorOutMin=[]  IntegratorOutMax=[]  FilterOutMin=[]  FilterOutMax=[]  SumI1OutMin=[]  SumI1OutMax=[]  SumI2OutMin=[]  SumI2OutMax=[]  SumI3OutMin=[]  SumI3OutMax=[]  SumI4OutMin=[]  SumI4OutMax=[]  SumDOutMin=[]  SumDOutMax=[]  DifferentiatorOutMin=[]  DifferentiatorOutMax=[]  FilterDiffOutCoefMin=[]  FilterDiffOutCoefMax=[]  ReciprocalOutMin=[]  ReciprocalOutMax=[]  SumDenOutMin=[]  SumDenOutMax=[]  SumNumOutMin=[]  SumNumOutMax=[]  DivideOutMin=[]  DivideOutMax=[]  UdiffTsProdOutMin=[]  UdiffTsProdOutMax=[]  NTsProdOutMin=[]  NTsProdOutMax=[]  UintegralTsProdOutMin=[]  UintegralTsProdOutMax=[]  UngainTsProdOutMin=[]  UngainTsProdOutMax=[]  ClampingZeroOutDataTypeStr=Inherit: Inherit via back propagation  ClampingZeroOutMin=[]  ClampingZeroOutMax=[]  FilterDenConstantOutDataTypeStr=Inherit: Inherit via back propagation  FilterDenConstantOutMin=[]  FilterDenConstantOutMax=[]  PCopyOutDataTypeStr=Inherit: Inherit via back propagation  PCopyOutMin=[]  PCopyOutMax=[]  NCopyOutDataTypeStr=Inherit: Inherit via back propagation  NCopyOutMin=[]  NCopyOutMax=[]  IntegratorContinuousStateAttributes=''  IntegratorStateMustResolveToSignalObject=off  IntegratorRTWStateStorageClass=Auto  FilterContinuousStateAttributes=''  FilterStateMustResolveToSignalObject=off  FilterRTWStateStorageClass=Auto  ParallelPVariant=InternalParameters  IdealPVariant=Disabled  IVariant=InternalParameters  DVariant=Disabled  IntegratorVariant=Continuous  SatVariant=Enabled  AWVariant=Passthrough  PCopyVariant=Disabled  TRVariant=Disabled  FdbkBlocksVariant=Forward  IdealPFdbkVariant=Disabled  SatFdbkVariant=Disabled  DerivativeFilterVariant=Disabled  NVariant=Disabled  NCopyVariant=Disabled_SignalSpec  FilterICVariant=Disabled  IntegratorICVariant=InternalICs  ExternalResetVariant=Disabled  TRSumVariant=Passthrough  SumFdbkVariant=Disabled  SumVariant=Sum_PI  TsampFilterVariant=InternalTs  TsampNgainVariant=Passthrough  TsampIntegralVariant=Passthrough  ExternalSaturationOutDataTypeStr=Inherit: Same as second input
  Power : Scope  Commented=on
  Power1 : Scope  Commented=on
  Product{,2..3,5} (4 alike) : Product  Commented=on
  Product1 : Product
  Product4 : Product
  R_battery : spsSeriesRLCBranchLib/Series RLC Branch  LConnTagsString=__new0  RConnTagsString=__new0  BranchType=R  Resistance=0.1  Inductance=1e-3  SetiL0=off  InitialCurrent=0  Capacitance=1440e-6  Setx0=off  InitialVoltage=80  Measurements=None
  S1_merge2 : Merge  Inputs=3  InitialOutput=[0]
  S2_merge2 : Merge  Inputs=3  InitialOutput=[0]
  S3_merge2 : Merge  Inputs=3  InitialOutput=[0]
  S4_merge2 : Merge  Inputs=3  InitialOutput=[0]
  Saturation{,2,4..5} (4 alike) : Saturate  Commented=on  UpperLimit=10  LowerLimit=-10
  Saturation1 : Saturate  Commented=on  UpperLimit=10  LowerLimit=-10  LinearizeAsGain=off
  Saturation3 : Saturate  Commented=on  UpperLimit=10  LowerLimit=-10  LinearizeAsGain=off
  Step2 : Step  Commented=on  Time=0.3  Before=5  After=5  SampleTime=0
  Step5 : Step  Commented=on  Time=0.3  Before=29  After=5  SampleTime=0
  Sum{,1..6} (7 alike) : Sum  Commented=on  Inputs=|+-
  Switch : Switch  Commented=on  Criteria=u2 > Threshold  SaturateOnIntegerOverflow=off  InputSameDT=off
  Terminator{,1..3} (4 alike) : Terminator
  Triangle Generator3 : spsTriangleGeneratorLib/Triangle Generator  Freq=wave_freq  Phase=0  Ts=0
  Triangle Generator4 : spsTriangleGeneratorLib/Triangle Generator  Freq=wave_freq  Phase=0  Ts=0
  VE : spsVoltageMeasurementLib/Voltage Measurement  PhasorSimulation=off  OutputType=Complex  PSBequivalent=0
  VE1 : spsVoltageMeasurementLib/Voltage Measurement  PhasorSimulation=off  OutputType=Complex  PSBequivalent=0
  VE2 : spsVoltageMeasurementLib/Voltage Measurement  PhasorSimulation=off  OutputType=Complex  PSBequivalent=0
  V_bus : Scope
  Vdc 1 : Scope  NumInputPorts=4
  Vdc 5 : Scope  NumInputPorts=6
  iL_ref : Scope
  iL_ref_merge2 : Merge  Inputs=3  InitialOutput=[0]
  max_load : Constant  Value=P_100
  mid_L : spsSeriesRLCBranchLib/Series RLC Branch  LConnTagsString=__new0  RConnTagsString=__new0  BranchType=L  Resistance=1.0  Inductance=40e-6  SetiL0=off  InitialCurrent=10  Capacitance=1.0  Setx0=off  InitialVoltage=0  Measurements=None
  mid_R : spsSeriesRLCBranchLib/Series RLC Branch  LConnTagsString=__new0  RConnTagsString=__new0  BranchType=R  Resistance=0.004  Inductance=1e-3  SetiL0=off  InitialCurrent=0  Capacitance=1e-3  Setx0=off  InitialVoltage=80  Measurements=None
  mode_selection : Scope  NumInputPorts=3
  u1_merge1 : Merge  Inputs=3  InitialOutput=[0]
  u2_merge2 : Merge  Inputs=3  InitialOutput=[0]
  + : PMIOPort  Tag=PMCPort  Side=Right
  - : PMIOPort  Tag=PMCPort  Port=2  Side=Right
  wires:
  Bus Selector/1 -> [Battery_SOC]  "<SOC (%)>"
  "85 volts, 100 Ah LithiumIon battery "/1 -> Bus Selector/1
  [S2] -> IGBT/Diode2/1
  [S1] -> IGBT/Diode1/1  "S1"
  [S1] -> Vdc 1/1  "S1"
  [S2] -> Vdc 1/2  "S2"
  [S3] -> Vdc 1/3  "S3"
  [S4] -> Vdc 1/4  "S4"
  Current Measurement/1 -> [iL]
  [S3] -> IGBT/Diode3/1
  [S4] -> IGBT/Diode4/1
  Sum/1 -> PID Controller2/1
  PID Controller2/1 -> Goto2/1
  From9/1 -> MATLAB Function/1(iL_ref)
  From10/1 -> MATLAB Function/2(iL)
  From12/1 -> MATLAB Function/3(vc_ref)
  From13/1 -> MATLAB Function/4(vc)
  From14/1 -> MATLAB Function/5(vin)
  From18/1 -> MATLAB Function/7(Ts)
  From96/1 -> MATLAB Function/6(i_out)
  From16/1 -> Modulation/1(u1)
  From17/1 -> Modulation/2(u2)
  Modulation/1(S1) -> Goto8/1
  Modulation/3(S3) -> Goto9/1
  Modulation/4(S4) -> Goto10/1
  Modulation/2(S2) -> Goto11/1
  Constant1/1 -> [Ts]
  [V_battery] -> Discharge+V/1  "Vin"
  Mux/1 -> Discharge+V/2  "iL"
  [iL_ref] -> Mux/2  "iL*"
  [iL] -> Mux/1  "iL"
  [V_bus] -> Mux1/1  "V_bus"
  [VC_ref] -> Mux1/2  "VC_ref"
  Mux1/1 -> Discharge+V/3  "V_out"
  Mux2/1 -> Discharge+V/6  "u1,u2"
  [u1] -> Mux2/1
  [u2] -> Mux2/2
  IGBT/Diode1/1 -> Terminator/1
  IGBT/Diode2/1 -> Terminator1/1
  IGBT/Diode4/1 -> Terminator2/1
  IGBT/Diode3/1 -> Terminator3/1
  VE1/1 -> [V_bus], V_bus/1
  MATLAB Function/2(u2) -> Saturation1/1
  MATLAB Function/1(u1) -> Saturation/1
  [i_out] -> Discharge+V/4  "i_output"
  [i_battery] -> Discharge+V/5  "i_battery"
  From11/1 -> Sum/1
  From28/1 -> Product/1  "Vc"
  From29/1 -> Product/2  "io"
  Product/1 -> Power/1
  From8/1 -> Sum/2
  From30/1 -> MATLAB Function1/2(iL)
  From55/1 -> MATLAB Function1/4(i_out)
  From36/1 -> MATLAB Function1/1(iL_ref)
  From37/1 -> MATLAB Function1/3(i_out_ref)
  From33/1 -> MATLAB Function1/5(vin)
  MATLAB Function1/1(u1) -> Saturation4/1
  From35/1 -> MATLAB Function1/7(Ts)
  MATLAB Function1/2(u2) -> Saturation5/1
  From38/1 -> Sum1/1
  Sum1/1 -> PID Controller1/1
  From31/1 -> Sum1/2
  PID Controller1/1 -> Goto20/1
  Modulation1/4(S4) -> Goto21/1
  Modulation1/1(S1) -> Goto23/1
  From40/1 -> Modulation1/2(u2)
  Modulation1/2(S2) -> Goto22/1
  Modulation1/3(S3) -> Goto24/1
  From39/1 -> Modulation1/1(u1)
  From52/1 -> MATLAB Function1/6(Vc)
  From62/1 -> Modulation2/2(u2)
  From61/1 -> Modulation2/1(u1)
  Modulation2/3(S3) -> Goto31/1
  Modulation2/4(S4) -> Goto30/1
  Modulation2/1(S1) -> Goto32/1
  Modulation2/2(S2) -> Goto29/1
  IL6/1 -> [i_battery]
  From53/1 -> MATLAB Function2/5(vin)
  From74/1 -> Gain2/1
  From59/1 -> MATLAB Function2/6(Vc)
  From58/1 -> Sum2/1
  From57/1 -> MATLAB Function2/3(i_out_ref)
  PID Controller3/1 -> Goto27/1
  Sum2/1 -> PID Controller3/1
  From54/1 -> MATLAB Function2/7(Ts)
  MATLAB Function2/1(u1) -> Goto15/1
  From56/1 -> MATLAB Function2/1(iL_ref)
  MATLAB Function2/2(u2) -> Goto25/1
  From34/1 -> Gain3/1
  Step2/1 -> Goto26/1
  From32/1 -> Gain/1
  Gain/1 -> MATLAB Function2/2(iL)
  Gain2/1 -> Sum2/2
  Gain3/1 -> MATLAB Function2/4(i_out)
  [VC_ref] -> Mux10/2  "VC_ref"
  [iL] -> Gain8/1  "iL"
  [V_battery] -> Mux10/1  "V_battery"
  Mux11/1 -> Vdc 5/6  "u1,u2"
  From94/1 -> Sum3/2
  From80/1 -> Modulation3/1(u1)
  [iL_ref] -> Mux9/2  "iL*"
  Mux9/1 -> Vdc 5/2  "iL"
  [u2] -> Mux11/2
  [V_bus] -> Vdc 5/1  "V_bus"
  PID Controller4/1 -> Goto36/1
  [u1] -> Mux11/1
  From81/1 -> Modulation3/2(u2)
  Mux10/1 -> Vdc 5/3  "V_out"
  From75/1 -> Sum3/1
  Sum3/1 -> PID Controller4/1
  Modulation3/1(S1) -> Goto41/1
  Modulation3/2(S2) -> Goto28/1
  Modulation3/3(S3) -> Goto40/1
  Modulation3/4(S4) -> Goto33/1
  Gain8/1 -> Mux9/1
  [i_out] -> Vdc 5/4  "i_bus"
  From95/1 -> Gain6/1
  From24/1 -> Gain10/1
  From70/1 -> MATLAB Function3/3(vc_ref)
  From76/1 -> MATLAB Function3/5(vin)
  MATLAB Function3/1(u1) -> Goto6/1
  From77/1 -> MATLAB Function3/4(vc)
  MATLAB Function3/2(u2) -> Goto7/1
  From78/1 -> MATLAB Function3/7(Ts)
  Gain6/1 -> MATLAB Function3/6(i_out)
  Gain10/1 -> MATLAB Function3/2(iL)
  Constant20/1 -> Goto37/1
  From79/1 -> MATLAB Function3/1(iL_ref)
  VE2/1 -> [V_battery_actual]
  From174/1 -> Sum5/1
  From193/1 -> Sum5/2
  PID Controller6/1 -> Goto91/1
  Sum5/1 -> PID Controller6/1
  Constant10/1 -> [Power_ref]
  Mux16/1 -> Discharge/3  "Power"
  Mux17/1 -> Discharge/6  "u1,u2"
  [Power_ref] -> Mux16/2
  Mux15/1 -> Discharge/2  "iL"
  [V_battery] -> Discharge/1  "V_battery"
  [iL] -> Mux15/1
  [Power_bus] -> Mux16/1
  [iL_ref] -> Mux15/2  "iL*"
  [u1] -> Mux17/1
  From188/1 -> Divide/1
  From189/1 -> Divide/2
  Divide/1 -> Goto96/1
  From171/1 -> MATLAB Function5/1(iL_ref)
  MATLAB Function5/2(u2) -> Goto89/1
  From173/1 -> Modulation5/1(u1)
  From172/1 -> MATLAB Function5/3(i_out_ref)
  From192/1 -> MATLAB Function5/4(i_out)
  Modulation5/1(S1) -> Goto94/1
  MATLAB Function5/1(u1) -> Goto88/1
  From175/1 -> Modulation5/2(u2)
  From169/1 -> MATLAB Function5/5(vin)
  Modulation5/2(S2) -> Goto93/1
  From168/1 -> MATLAB Function5/2(iL)
  From170/1 -> MATLAB Function5/7(Ts)
  Modulation5/4(S4) -> Goto92/1
  Modulation5/3(S3) -> Goto95/1
  From191/1 -> MATLAB Function5/6(Vc)
  [V_bus] -> Mux18/1  "V_bus"
  Mux18/1 -> Discharge/4  "V_out"
  [VC_ref] -> Mux18/2
  [i_out] -> Mux19/1  "i_bus"
  [i_out_ref] -> Mux19/2  "i_ref"
  Mux19/1 -> Discharge/5  "i_out"
  [u2] -> Mux17/2
  Constant5/1 -> Goto38/1
  Divide1/1 -> Goto46/1
  From101/1 -> Sum4/1
  Constant12/1 -> Goto100/1
  PID Controller5/1 -> Goto39/1
  Product2/1 -> ActualPower1/1, Goto99/1
  From107/1 -> Gain12/1
  From103/1 -> Divide1/1
  From104/1 -> Product2/1, Divide1/2
  Sum4/1 -> PID Controller5/1
  Mux14/1 -> Charge/6  "u1,u2"
  [u2] -> Mux14/2
  [i_battery] -> Mux21/1  "i_bus"
  [i_out_ref] -> Gain15/1  "i_ref"
  [V_bus] -> Charge/1  "V_in"
  Mux21/1 -> Charge/5  "i_out"
  [V_charge_PowerMode] -> Mux20/2
  [u1] -> Mux14/1
  Mux12/1 -> Charge/2  "iL"
  [Power_battery] -> Mux13/1
  Mux13/1 -> Charge/3  "Power"
  Mux20/1 -> Charge/4  "V_battery"
  [Power_ref] -> Gain7/1
  [iL_ref] -> Gain14/1  "iL*"
  From198/1 -> Gain11/1
  Gain11/1 -> Sum4/2
  [iL] -> Mux12/1
  [V_battery] -> Mux20/1
  Gain16/1 -> MATLAB Function6/2(iL)
  MATLAB Function6/2(u2) -> Goto102/1
  From200/1 -> MATLAB Function6/7(Ts)
  From202/1 -> MATLAB Function6/3(i_out_ref)
  From190/1 -> Gain16/1
  From201/1 -> MATLAB Function6/1(iL_ref)
  From199/1 -> MATLAB Function6/5(vin)
  From197/1 -> Gain17/1
  MATLAB Function6/1(u1) -> Goto101/1
  From203/1 -> MATLAB Function6/6(Vc)
  Gain17/1 -> MATLAB Function6/4(i_out)
  Modulation6/3(S3) -> Goto103/1
  From93/1 -> Modulation6/2(u2)
  Modulation6/2(S2) -> Goto34/1
  Modulation6/1(S1) -> Goto104/1
  Modulation6/4(S4) -> Goto35/1
  From64/1 -> Modulation6/1(u1)
  Gain12/1 -> Product2/2
  [V_bus] -> Product4/1
  Product4/1 -> BusPower/1, [Power_bus]
  [i_out] -> Product4/2
  Constant14/1 -> Goto126/1
  From41/1 -> BatteryCurrent1/1
  Product1/1 -> ActualPower2/1, [Power_battery]
  [V_battery] -> Product1/1
  [i_battery] -> Product1/2
  Constant16/1 -> [V_charge_PowerMode]
  Gain7/1 -> Mux13/2
  Gain15/1 -> Mux21/2
  Gain14/1 -> Mux12/2
  u1_merge1/1 -> [u1]
  iL_ref_merge2/1 -> [iL_ref]
  u2_merge2/1 -> [u2]
  S4_merge2/1 -> [S4]
  S1_merge2/1 -> [S1]
  S3_merge2/1 -> [S3]
  S2_merge2/1 -> [S2]
  [S1_D] -> S1_merge2/1
  [S2_D] -> S2_merge2/1
  [S3_D] -> S3_merge2/1
  [S4_D] -> S4_merge2/1
  [iL_ref_D] -> iL_ref_merge2/1
  [u1_D] -> u1_merge1/1
  [u2_D] -> u2_merge2/1
  [S1_C] -> S1_merge2/2
  [S2_C] -> S2_merge2/2
  [S3_C] -> S3_merge2/2
  [S4_C] -> S4_merge2/2
  [iL_ref_C] -> iL_ref_merge2/2
  [u1_C] -> u1_merge1/2
  [u2_C] -> u2_merge2/2
  From92/1 -> Product3/2  "io"
  From45/1 -> Sum6/1
  From88/1 -> Product3/1  "Vc"
  Modulation4/1(S1) -> Goto77/1
  Modulation4/4(S4) -> Goto42/1
  From49/1 -> Modulation4/1(u1)
  From50/1 -> Modulation4/2(u2)
  PID Controller7/1 -> Goto75/1
  Sum6/1 -> PID Controller7/1
  Modulation4/3(S3) -> Goto78/1
  From98/1 -> Sum6/2
  Product3/1 -> Power1/1
  Modulation4/2(S2) -> Goto43/1
  Constant4/1 -> Goto80/1
  VE/1 -> [V_battery]
  Saturation/1 -> Goto12/1
  Saturation1/1 -> Goto14/1
  [iL] -> Charge Mixed CurrentPower1/2(iL)
  [Ts] -> Discharge Const Voltage/5(TimeStep)
  Charge Mixed CurrentPower1/1(S1) -> [S1_C]
  Triangle Generator3/1 -> Discharge Const Voltage/6(Triangular_generator)
  Charge Mixed CurrentPower1/3(S3) -> [S3_C]
  Charge Mixed CurrentPower1/6(u1) -> [u1_C]
  [V_battery] -> Charge Mixed CurrentPower1/3(V_battery)
  Charge Mixed CurrentPower1/2(S2) -> [S2_C]
  [i_out_ref] -> Charge Mixed CurrentPower1/6(i_out_ref)
  If1/2 -> Charge Mixed CurrentPower1/Action
  [Ts] -> Charge Mixed CurrentPower1/5(TimeStep)
  Triangle Generator4/1 -> Charge Mixed CurrentPower1/7(Triangular_generator)
  Charge Mixed CurrentPower1/4(S4) -> [S4_C]
  [i_out] -> Discharge Const Voltage/4(I_out)
  Discharge Const Voltage/1(S1) -> [S1_D]
  Discharge Const Voltage/3(S3) -> [S3_D]
  [V_bus] -> Charge Mixed CurrentPower1/1(V_bus)
  Charge Mixed CurrentPower1/7(u2) -> [u2_C]
  Discharge Const Voltage/2(S2) -> [S2_D]
  Charge Mixed CurrentPower1/5(iL_ref) -> [iL_ref_C]
  [V_battery] -> Discharge Const Voltage/3(V_battery)
  Discharge Const Voltage/5(iL_ref) -> [iL_ref_D]
  Discharge Const Voltage/6(u1) -> [u1_D]
  Discharge Const Voltage/7(u2) -> [u2_D]
  [discharge_signal] -> MATLAB Function4/1(discharge_mode_flag), mode_selection/1, If1/1  "u1"
  [i_battery] -> Charge Mixed CurrentPower1/4(I_battery)
  [V_bus] -> Discharge Const Voltage/1(V_bus)
  [iL] -> Discharge Const Voltage/2(iL)
  If1/4 -> DoNothing2/Action
  If1/1 -> Discharge Const Voltage/Action
  Discharge Const Voltage/4(S4) -> [S4_D]
  [VC_ref] -> Discharge Const Voltage/7(V_bus_ref)
  [V_battery_actual] -> Divide3/1
  Divide3/1 -> Battery Load/1  "Battery_load"
  [i_battery] -> Divide3/2
  From148/1 -> MATLAB Function/8(Bus_load)
  Current Measurement1/1 -> I_bus_scope/1, [i_out]
  From156/1 -> MATLAB Function7/8(Bus_load)
  MATLAB Function7/1(u1) -> Saturation2/1
  Saturation3/1 -> Goto119/1
  Saturation2/1 -> Goto81/1
  MATLAB Function7/2(u2) -> Saturation3/1
  From154/1 -> MATLAB Function7/4(vc)
  From155/1 -> MATLAB Function7/5(vin)
  From158/1 -> MATLAB Function7/1(iL_ref)
  From152/1 -> MATLAB Function7/2(iL)
  From157/1 -> MATLAB Function7/7(Ts)
  From153/1 -> MATLAB Function7/3(vc_ref)
  From159/1 -> MATLAB Function7/6(i_out)
  Constant11/1 -> Goto120/1
  Switch/1 -> Goto76/1
  From47/1 -> Switch/3
  From48/1 -> Product5/1
  From51/1 -> Product5/2
  Product5/1 -> Switch/1
  From46/1 -> Minus/1
  From44/1 -> Minus/2
  [VC_ref] -> iL_ref/1  "iL*"
  Minus/1 -> Switch/2
  [Bus_load] -> Discharge Const Voltage/8(Bus_load)
  Step5/1 -> Goto19/1
  Saturation4/1 -> Goto17/1
  Saturation5/1 -> Goto18/1
  [Battery_SOC] -> If1/2, mode_selection/2  "u2"
  [V_battery] -> MATLAB Function4/2(v_battery)
  [V_bus] -> MATLAB Function4/3(v_bus)
  [i_battery] -> MATLAB Function4/4(i_battery)
  [i_out] -> MATLAB Function4/5(i_bus)
  If1/3 -> Charge Mixed CurrentPower2/Action
  Charge Mixed CurrentPower2/7(u2) -> [u2_protect]
  Charge Mixed CurrentPower2/1(S1) -> [S1_protect]
  Charge Mixed CurrentPower2/6(u1) -> [u1_protect]
  Charge Mixed CurrentPower2/5(iL_ref) -> [iL_ref_protect]
  Charge Mixed CurrentPower2/3(S3) -> [S3_protect]
  Charge Mixed CurrentPower2/2(S2) -> [S2_protect]
  Charge Mixed CurrentPower2/4(S4) -> [S4_protect]
  [S1_protect] -> S1_merge2/3
  [S2_protect] -> S2_merge2/3
  [S3_protect] -> S3_merge2/3
  [S4_protect] -> S4_merge2/3
  [iL_ref_protect] -> iL_ref_merge2/3
  [u1_protect] -> u1_merge1/3
  [u2_protect] -> u2_merge2/3
  MATLAB Function4/1(block_status) -> Cast To Double/1
  Cast To Double/1 -> If1/3, mode_selection/3  "u3"
  [i_out_ref] -> Mux3/2
  Mux3/1 -> Vdc 5/5  "i_battery"
  [i_battery] -> Mux3/1  "i_battery"
  [Battery_SOC] -> Battery Load/2
  [V_battery_actual] -> Mux4/1
  [V_battery] -> Mux4/2
  Mux4/1 -> Battery Load/4  "V_out"
  [i_battery] -> Battery Load/3
  battery_I_charge_ref/1 -> [i_out_ref]
  V_bus_ref/1 -> [VC_ref]
  From60/1 -> MATLAB Function/9(i_battery)
  [i_battery] -> Discharge Const Voltage/9(i_battery)
  Bus_load/1 -> [Bus_load]
  Mode=Charge0/DIscharge1/1 -> [discharge_signal]
  From43/1 -> MATLAB Function/10(P_full_load)
  max_load/1 -> [Power_max]
  [Power_max] -> Discharge Const Voltage/10(Power_full)
  connections:
  "85 volts, 100 Ah LithiumIon battery "/LConn2 -- VE2/LConn2 -- R_battery/LConn1
  IGBT/Diode1/RConn1 -- mid_R/RConn1 -- IGBT/Diode2/LConn1
  IGBT/Diode4/LConn1 -- Current Measurement/RConn1 -- IGBT/Diode3/RConn1
  mid_L/RConn1 -- Current Measurement/LConn1
  mid_R/LConn1 -- mid_L/LConn1
  Current Measurement1/RConn1 -- VE1/LConn1 -- +/RConn1
  IL6/LConn1 -- VE2/LConn1 -- "85 volts, 100 Ah LithiumIon battery "/LConn1
  C1/LConn1 -- DM_inductor1/RConn1 -- VE/LConn1 -- IGBT/Diode1/LConn1
  R_battery/RConn1 -- VE/LConn2 -- -/RConn1 -- VE1/LConn2 -- C2/RConn1 -- IGBT/Diode4/RConn1 -- IGBT/Diode2/RConn1 -- C1/RConn1
  C2/LConn1 -- DM_inductor2/LConn1 -- IGBT/Diode3/LConn1
  IL6/RConn1 -- DM_inductor1/LConn1
  DM_inductor2/RConn1 -- Current Measurement1/LConn1

== system rectifire_single_inverter_pv1/inverter/Subsystem ==
  Udc : Inport
  Constant : Constant  Value=350
  Discrete PI Controller : powerlib_extras/Discrete  Control Blocks/Discrete PI Controller  Kp=2  Ki=50  Par_Limits=[1e6 -1e6]  Init=0  Ts=2e-7
  Logical Operator2 : Logic  Operator=NOT  AllPortsSameDT=off  OutDataTypeStr=boolean
  PWM1 : Subsystem
  Repeating Sequne2 : simulink/Sources/Repeating Sequence  rep_seq_t=[0 5e-6 10e-6 15e-6 20e-6]  rep_seq_y=[0 1 0 -1 0]
  Scope11 : Scope
  Scope12 : Scope
  Sum5 : Sum  Inputs=|+-
  DC_PWM2 : Outport
  DC_PWM1 : Outport  Port=2
  wires:
  Discrete PI Controller/1 -> Scope12/1, PWM1/1(In1)
  PWM1/1(Out1) -> DC_PWM1/1, Logical Operator2/1
  Sum5/1 -> Scope11/1, Discrete PI Controller/1
  Repeating Sequne2/1 -> PWM1/2(In2)
  Udc/1 -> Sum5/1
  Constant/1 -> Sum5/2
  Logical Operator2/1 -> DC_PWM2/1

== system rectifire_single_inverter_pv1/motor/Anti_Park ==
  Vd : Inport
  thetam : Inport  Port=2
  Vq : Inport  Port=3
  Fcn : Fcn  Expr=cos(u[1])*u[2]-sin(u[1])*u[3]
  Fcn1 : Fcn  Expr=sin(u[1])*u[2]+cos(u[1])*u[3]
  Mux1 : Mux  Inputs=3
  Ualpha : Outport  VectorParamsAs1DForOutWhenUnconnected=off
  Ubeta : Outport  Port=2  VectorParamsAs1DForOutWhenUnconnected=off
  wires:
  Fcn1/1 -> Ubeta/1
  Fcn/1 -> Ualpha/1
  Mux1/1 -> Fcn/1, Fcn1/1
  Vd/1 -> Mux1/2
  Vq/1 -> Mux1/3
  thetam/1 -> Mux1/1

== system rectifire_single_inverter_pv1/motor/Clark ==
  A : Inport
  B : Inport  Port=2
  C : Inport  Port=3
  Mux : Mux  Inputs=3
  alpha : Fcn  Expr=(u(1)-0.5*(u(2)+u(3)))*2/3
  beta : Fcn  Expr=sqrt(3)/2*(u(2)-u(3))*2/3
  Alpha : Outport  VectorParamsAs1DForOutWhenUnconnected=off
  Beta : Outport  Port=2  VectorParamsAs1DForOutWhenUnconnected=off
  wires:
  alpha/1 -> Alpha/1
  B/1 -> Mux/2
  C/1 -> Mux/3
  A/1 -> Mux/1
  Mux/1 -> beta/1, alpha/1
  beta/1 -> Beta/1

== system rectifire_single_inverter_pv1/motor/Park ==
  Alpha : Inport
  Beta : Inport  Port=2
  The : Inport  Port=3
  Mux : Mux  Inputs=3
  Transfer Fcn : TransferFcn  Denominator=[0.002 1]
  Transfer Fcn1 : TransferFcn  Denominator=[0.002 1]
  d : Fcn  Expr=u(1)*cos(u(3))+u(2)*sin(u(3))
  q : Fcn  Expr=-u(1)*sin(u(3))+u(2)*cos(u(3))
  D : Outport  VectorParamsAs1DForOutWhenUnconnected=off
  Q : Outport  Port=2  VectorParamsAs1DForOutWhenUnconnected=off
  wires:
  Beta/1 -> Mux/2
  Alpha/1 -> Mux/1
  Mux/1 -> q/1, d/1
  The/1 -> Mux/3
  d/1 -> D/1
  q/1 -> Q/1
